simulink model "LowPassFilter"  (R2021b)
settings: Solver=VariableStepAuto  StartTime=0.0  StopTime=10.0  RelTol=1e-3
libraries: simulink x1
settings Model: Creator=hp  LastModifiedBy=hp

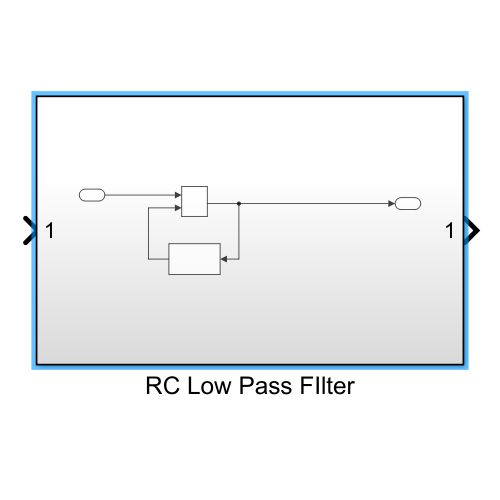
[thumbnail: Simulink's stored preview of the top-level diagram]
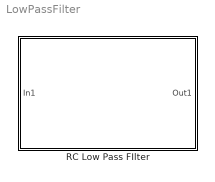
== system LowPassFilter ==
  RC Low Pass FIlter : Subsystem

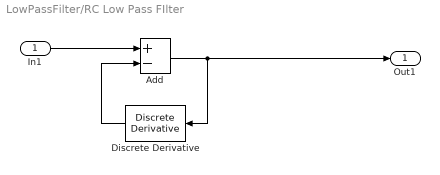
== system LowPassFilter/RC Low Pass FIlter ==
  In1 : Inport
  Add : Sum  Inputs=||+||-||
  Discrete Derivative : simulink/Discrete/Discrete Derivative  gainval=1  ICPrevScaledInput=0.0  OutMin=[]  OutMax=[]  OutDataType=fixdt(1, 16)  OutScaling=2^-10  DoSatur=off
  Out1 : Outport
  wires:
  In1/1 -> Add/1
  Add/1 -> Discrete Derivative/1, Out1/1
  Discrete Derivative/1 -> Add/2
